simulink library "mympclib"  (R2020a)
settings: Solver=VariableStepAuto  StartTime=0.0  StopTime=10.0  RelTol=1e-3
undefined symbols (not defined in the file): params, sysm, Ts
(part 1 of 2)
settings Model: Creator=kohei  LastModifiedBy=kohei

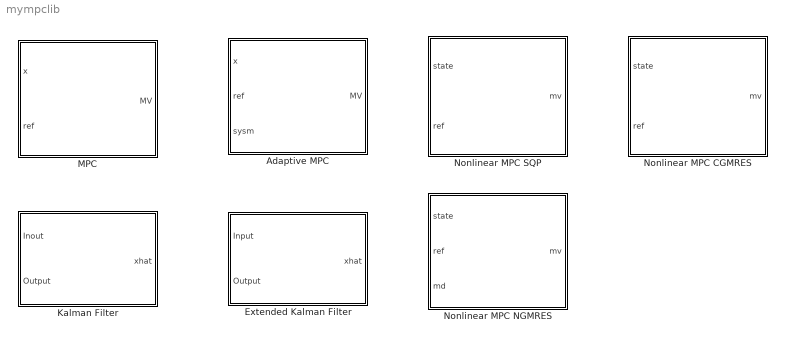
== system mympclib ==
  Adaptive MPC : Subsystem  TreatAsAtomicUnit=on  mask(Adaptive Model Predictive Control){params=params, numState=1, numRef=1, numMV=1, Ts=Ts, enableDist=off, numDist=1, enableSlack=off, enableStatus=off, enableMVseq=off}
      mask prompts: params "MPC Parameters"; numState "Dimension of State"; numRef "Dimension of Reference"; numMV "Dimension of Input"; Ts "Sampling time"; enableDist "Enable Disturbance Input"; numDist "Dimension of Disturbance"; enableSlack "Enable Slack Output"; enableStatus "Enable Status Output"; enableMVseq "Enable MVseq Output"
      mask help:
      | This is the Adaptive MPC (AMPC) Controller.
      | AMPC calculates the QP problem based on the linear plant model.
      | If you want to see the description, please push the help button.
      mask init:
      | numDist = initMaskPortMPC(numDist,enableDist,enableSlack,enableStatus,enableMVseq,'Adaptive MPC');
      | [params,~] = initMaskMPC(params,[],numState,numRef,numMV,numDist,'Adaptive MPC');
      | index = numState*params.PredictiveHorizon;
      | index2 = numMV*params.ControlHorizon;
      | index3 = numRef*params.PredictiveHorizon;
      | index4 = numMV*params.ControlHorizon+1;
      | index5 = 4*(numMV*params.ControlHorizon)+2*(numRef*params.PredictiveHorizon)+1;
      mask Help:
      | This block is the Adaptive MPC Controller.
      | AMPC calculates the QP problem based on the linear plant model.
      | 
      | >>Optimization formulation
      | -------------------------------------------------------------------------------------------------------------------------------------------------------------------
      | This MPC is formulated based on the next QP optimization.
      | 
      | J = 0.5 * ( (y - yref)'*Q*(y - yref) + du'*R*du + rho*slack^2 )
      | 
      | Subject to :
      | umin <= u <= umax
      | dumin <= du <= dumax
      | ymin - slack*vmin <= y <= ymax + slack*vmax
      | skack >= 0
      | 
      | One slack varable is introduced for relaxing the output constraint.
      | The vmin and vmax are the tunable parameter for relaxation which is able to specified by MPC parameter structure as "params.softConstRelaxation".
      | Please read the " Details of the parameter sturucture "params" and "sysm" ".
      | -------------------------------------------------------------------------------------------------------------------------------------------------------------------
      | 
      | >> Model Structure
      | -------------------------------------------------------------------------------------------------------------------------------------------------------------------
      | This block supports the discrete plant system as shown bellow:
      | Uppercase is indicated the Nominal value, Lowercase with 'd' suffix is indicated the perturbation.
      | 
      | State : x = X + dx
      | MV : u = U + du
      | Measurement Disturbance(MD) : md = MD + dmd
      | Output Value : y = Y +dy (dy = C*dx)
      | 
      | Model formulation :
      | dx(k+1) = A*dx(k)+ B*du(k) + Bd*dmd(k) + f0
      | y(K) = C*dx(K) + Y
      | 
      | Note : The direct feedthrough term "D" is not considered in this system.
      |           "f0" is the nominal value of the system at the operation point.
      | 
      | The plant model is streamed from the Input port "sysm" which is the Bus signal.
      | You need to define the Bus object named "sysBus" which includes A, B, Bd, C, f0 vector/matrix and the operation point of state, input, disturbance and output.
      | -------------------------------------------------------------------------------------------------------------------------------------------------------------------
      | 
      | >>Parameter
      | -------------------------------------------------------------------------------------------------------------------------------------------------------------------
      | The MPC parameter must be defined as structure variable.
      | And you must need to clarify the each dimension of "state", "ref", and "Input" and the Sampling time through mask dialog.
      | 
      | This block has four input ports "state", "ref", "md" and "sysm".
      | Where "n" is the order of state, "l" is the order of output value (OV), "m" is the order of manipulated variable (MV) and "nd" is the order of measurement disturbance (MD).
      | "state" : State variable of plant model (n×1)
      | "ref" : Reference for OV  (l×1)
      | "md" : Measurement Disturbance (nd×1)
      | "sysm" : Bus signal which includes the predictive model. The structuer of the Bus object is shown bellow :
      | 
      | sysm.A : A matrix
      | sysm.B : B matrix for MV
      | sysm.Bd : B matrix for MD
      | sysm.C : C matrix
      | sysm.U : Operation point of MV, Defalt : zeros(m,1)
      | sysm.MD : Operation point of MD, Default : zeros(nd,1)
      | sysm.Y : Operation point of OV, Default : zeros(l,1)
      | sysm.X : Operation point of state, Default : zeros(n,1)
      | sysm.f0: Operation point of system, Default : zeros(n,1)
      | 
      | You can create a Bus object automatically by uisng the API "createSysBusObject".
      | The API has four arguments 'n, m, nd, l'.
      | Example :
      | >sysBus = createSysBusObject(n,m,nd,l)
      | 
      | The output is four "mv" , "slack", "status" and "mvseq".
      | "mv" : Manipulated Variable which is optimized by MPC. (m×1)
      | "slack" : Slack variable for softening OV constrain. This value must be grater than 0 (>= 0).
      |              If the value is grater than 0, the OV constraint is softed to avoid infeasibe.
      | "status" : Status is for seeing whether or not feasible . If the value is "1", it means feasible, on the other hand the value is 0, it means infeasible.
      |                When the status is "0", the MPC applies a last MV for current step.
      | "mvseq": Sequence value of MV for futuer
      | -------------------------------------------------------------------------------------------------------------------------------------------------------------------
      | 
      | >>Solver
      | -------------------------------------------------------------------------------------------------------------------------------------------------------------------
      | You can choose two types solver for solving the QP.
      | First is the "Active set".
      | Second is the "Interior Point Method".
      | 
      | The Active set is appropriate to optimization class for small or middle size.
      | The Interior Point Method is appropriate to optimization class for large size.
      | 
      | Both default max iteration number is 50.
      | -------------------------------------------------------------------------------------------------------------------------------------------------------------------
      | 
      | >>Details of the parameter sturucture "params" and "sysm"
      | -------------------------------------------------------------------------------------------------------------------------------------------------------------------
      | The MPC parameter sturucture "params" must be configured as shown bellow :
      | Where "n" is the order of state, "l" is the order of OV, "m" is the order of MV and the "nd" is the order of MD.
      | 
      | params.Q : Weight of OV (l×l) , Default : Unit matrix
      | params.R : Weight of MV (m×m), Default : Unit matrix
      | params.PredictiveHorizon : Predictive horizon (Scalar), Default : 10
      | params.Controlhorizon : Control Horizon (Scalar), Default : 5
      | params.MV_max : MV max (m×1), Default : 999
      | params.MV_min : MV min (m×1), Default :  -999
      | params.dMV_max : Rate of MV max (m×1), Default : 999
      | params.dMV_min : Rate of MV min(m×1), Default : -999
      | params.OV_max : Rate of OV max (l×1), Default : 999
      | params.OV_min : Rate of OV min (l×1), Default : -999
      | params.rho : Weight of slack variable (Scalar), Default : 10^4
      | params.softConstRelaxation : Constant for OV relaxation by slack variable (l×1), Default : ones(l,1)
      | params.MV_scalefactor : Scale gain for MV (m×1), Default : ones(m,1)
      | params.OV_scalefactor : Scale gain for OV (l×1), Default : ones(m,1)
      | params.MD_scalefactor : Scale gain for MD (nd×1), Default : ones(m,1)
      | params.initialconditionMV : Initial value for MV (m×1), Default : ones(m,1)
      | params.SolverType :Scalar 1:= Active Set, 2:= Interior Point Method, Default : 1 (Active set)
      | params.IterationMax : Max iteration number of the QP solver, Default : 50
      | -------------------------------------------------------------------------------------------------------------------------------------------------------------------
      | 
      | >>Code generation
      | -------------------------------------------------------------------------------------------------------------------------------------------------------------------
      | Yes, support. If you have Simulink Coder and Embedded Coder, the implementation code can be generated from this block.
      | -------------------------------------------------------------------------------------------------------------------------------------------------------------------
      mask Callback enableDist:
      | enab = get_param(gcb,'enableDist');
      | 
      | % Set the 'MaskVisibilities' property for each parameters
      | if strcmp(enab,'on')
      |     set_param(gcb,'MaskVisibilities',{'on','on','on','on','on','on','on','on','on','on'});
      | else
      |     set_param(gcb,'MaskVisibilities',{'on','on','on','on','on','on','off','on','on','on'});
      | end
      mask Display:
      | fprintf('Adaptive MPC')
      | port_label('Output', 1, 'mv')
      | port_label('Input', 1, 'state')
      | port_label('Input', 2, 'ref')
      | port_label('Input', 3, 'sysm')
  Extended Kalman Filter : Subsystem  TreatAsAtomicUnit=on  mask(Extended Kalman filter){stateFunction=0, jacobianStateFunction=0, measurementFunction=0, jacobianMeasurmentFunction=0, Bv=0, Q=0, R=0, xhat0=0, P0=0, Ts=0, numState=0, numOutput=0, enableP=off, enableG=off}
      mask prompts: stateFunction "State Function"; jacobianStateFunction "Jacobian for the State Function"; measurementFunction "Measurment Function"; jacobianMeasurmentFunction "Jacobian for the Measurement Function"; Bv "Matrix for System noise v"; Q "Covariance matrix Q for system noise v"; R "Covariance matrix R for measurement noise w"; xhat0 "Initial value for xhat which is column vector"; P0 "Initial value for covariance matrix P"; Ts "Sampling time Ts"; numState "Order of state"; numOutput "Order of output"; enableP "Enable Covariance Marix output"; enableG "Enable Kalman Gain Matrix"
      mask help: This is the Extended Kalman filter(EKF) block.
      mask init:
      | p = initMaskEKF(stateFunction,measurementFunction,jacobianStateFunction,jacobianMeasurmentFunction);
      | initMaskPortKF(enableP,enableG,'EKF')
      mask Help:
      | This is the Extended Kalman filter(EKF) block.
      | Some parametrs are set through the mask diagram.
      | This block has two inputs named "Input" and "Output".
      | And it has three outputs named "xhat (Estimated state)", "P (Covariance matrix )" and "G (Kalman gain matrix )".
      | 
      | Support Formulation of EKF :
      | x(k+1) = f(x(k),u(k)) + Bv*v(k)
      | y(k) = h(x(k),u(k)) + w(k)
      | 
      | n : Order of state
      | m : Order of input
      | l : Order of output
      | 
      | f : Nonlinear dynamics function (n,1)
      | h : Nonlinear measurement function (l,1)
      | Bv : Gain matrix Bv for system noise v (n,n)
      | x : State (n,1)
      | u : Input (m,1)
      | v: System noise (n,1)
      | y : Output (l,1)
      | w : Measurement noise (l,1)
      | 
      | You need to prepare four MATLAB function and put them on the current folder or the MATLAB path.
      | Kind of the MATLAB function :
      | 
      | >Nonlinear discrete state function
      | 
      | >Jacobian of the Nonlinear state function about the state x with operate conditions x0 and u0.
      | 
      | >Nonlinear measurement function
      | 
      | >Jacobian of the Nonlinear measurement function about the state x with operate conditions x0 and u0.
      | 
      | Where, the above functions must be accepted three arguments x(state), u(input) and Ts(sampling time), and one output.
      | The order of three arguments has to be put as state, input and sampling time such like a below:
      | 
      | function out = fcn(x, u, Ts)
      | 
      | You have to set these function names through this mask dialog as the character array  by using sigle quotation.
      mask Display:
      | fprintf('Extended\n Kalman Filter')
      | port_label('Output', 1, 'xhat')
      | port_label('Input', 1, 'Input')
      | port_label('Input', 2, 'Output')
  Kalman Filter : Subsystem  TreatAsAtomicUnit=on  mask(Kalman filter){A=0, Bu=0, Bv=0, C=0, Q=0, R=0, xhat0=0, P0=0, Ts=0, enableP=off, enableG=off}
      mask prompts: A "System matrix A"; Bu "Input matrix Bu"; Bv "System noise matrix Bv"; C "Measurement matrix C"; Q "Covariance matrix for System noise v"; R "Covariance matrix for Measurement noise w"; xhat0 "Initial value for xhat which is column vector"; P0 "Initial value for covariance matrix P"; Ts "Sampling time Ts"; enableP "Enable Covariance Marix output"; enableG "Enable Kalman Gain Matrix"
      mask help: This is the LTI Kalman filter block.
      mask init:
      | initMaskPortKF(enableP,enableG,'KF')
      mask Help:
      | This is the LTI Kalman filter block.
      | All parametrs are set through the mask diagram.
      | This block has two inputs named "Input" and "Output".
      | And it has three outputs named "xhat (Estimated state)", "P (Covariance matrix )" and "G (Kalman gain matrix )".
      | 
      | Support Formulation of Kalman filter :
      | x(k+1) = A*x(k) + Bu*u(k) + Bv*v(k)
      | y(k) = C*x(k) + w(k)
      | 
      | A : System matrix A for state
      | Bu : System matrix Bu for input u
      | Bv : Gain matrix Bv for system noise v
      | C : System matrix C for output
      | x : State
      | u : Input
      | v : System noise
      | y : Output
      | w : Measurement noise
      mask Display:
      | fprintf('Kamlman Filter')
      | port_label('Output', 1, 'xhat')
      | port_label('Input', 1, 'Input')
      | port_label('Input', 2, 'Output')
  MPC : Subsystem  TreatAsAtomicUnit=on  mask(Model Predictive control){params=params, sysm=sysm, numState=1, numRef=1, numMV=1, Ts=Ts, enableDist=off, numDist=1, enableSlack=off, enableStatus=off, enableMVseq=off}
      mask prompts: params "MPC Parameters"; sysm "Control system"; numState "Dimension of State"; numRef "Dimension of Reference"; numMV "Dimension of MV"; Ts "Sampling time"; enableDist "Enable Disturbance Input"; numDist "Dimension of Disturbance"; enableSlack "Enable Slack Output"; enableStatus "Enable Status Output"; enableMVseq "Enable MVseq Output"
      mask help:
      | This is the MPC Controller.
      | MPC calculates the QP problem based on the linear plant model.
      | If you want to see the description, please push the help button.
      mask init:
      | numDist = initMaskPortMPC(numDist,enableDist,enableSlack,enableStatus,enableMVseq,'MPC');
      | [params,sysm] = initMaskMPC(params,sysm,numState,numRef,numMV,numDist,'MPC');
      | index = numState*params.PredictiveHorizon;
      | index2 = numMV*params.ControlHorizon;
      | index3 = numRef*params.PredictiveHorizon;
      | index4 = numMV*params.ControlHorizon+1;
      | index5 = 4*(numMV*params.ControlHorizon)+2*(numRef*params.PredictiveHorizon)+1;
      mask Help:
      | This block is the MPC Controller.
      | MPC calculates the QP problem based on the linear plant model.
      | 
      | >>Optimization formulation
      | -------------------------------------------------------------------------------------------------------------------------------------------------------------------
      | This MPC is formulated based on the next QP optimization.
      | 
      | J = 0.5 * ( (y - yref)'*Q*(y - yref) + du'*R*du + rho*slack^2 )
      | 
      | Subject to :
      | umin <= u <= umax
      | dumin <= du <= dumax
      | ymin - slack*vmin <= y <= ymax + slack*vmax
      | skack >= 0
      | 
      | One slack varable is introduced for releaxing the output constraint.
      | The vmin and vmax are tunable parameters for relaxation which are specified by the MPC parameter structure as "params.softConstRelaxation".
      | Please read the " Details of the parameter sturucture "params" and "sysm" ".
      | -------------------------------------------------------------------------------------------------------------------------------------------------------------------
      | 
      | 
      | >> Model Structure
      | -------------------------------------------------------------------------------------------------------------------------------------------------------------------
      | This block supports the discrete plant system as shown bellow:
      | Uppercase is indicated the Nominal value, Lowercase with 'd' suffix is indicated the perturbation.
      | 
      | State : x = X + dx
      | MV : u = U + du
      | Measurement Disturbance(MD) : md = MD + dmd
      | Output Value : y = Y +dy (dy = C*dx)
      | 
      | Model formulation :
      | dx(k+1) = A*dx(k)+ B*du(k) + Bd*dmd(k) + f0
      | y(K) = C*dx(K) + Y
      | 
      | Note : The direct feedthrough term "D" is not considered in this system.
      |           "f0" is the nominal value of the system at the operation point.
      | -------------------------------------------------------------------------------------------------------------------------------------------------------------------
      | 
      | 
      | >>Parameter
      | -------------------------------------------------------------------------------------------------------------------------------------------------------------------
      | The MPC parameter and the Control system must be defined as a structure variable.
      | The Sampling time must be set through mask dialog.
      | 
      | This block has three input ports "state", "ref" and "md".
      | Where, "n" is the order of state, "l" is the order of Output value (OV),  "m" is the order of Manipulated variable (MV) and "nd" is the order of measurment disturbance (MD).
      | "state" : State variable of plant model (n×1)
      | "ref" : Reference for OV  (l×1)
      | "md" : Measurement Disturbance (nd×1)
      | 
      | The output is three "mv" , "slack" and "status".
      | "MV" : Manipulated Variable which is optimized by MPC. (m×1)
      | "slack" : Slack variable for softening OV constrain. This value must be grater than 0 (>= 0).
      |              If the value is grater than 0, the OV constraint is softed to avoid infeasibe.
      | "status" : Status is for seeing whether or not feasible. If the value is "1", it means feasible, on the other hand the value is "0", it means infeasible.
      |                When the status is "0", the MPC applies a last MV for current step.
      | "mvseq": Sequence value of MV for futuer
      | -------------------------------------------------------------------------------------------------------------------------------------------------------------------
      | 
      | >>Solver
      | -------------------------------------------------------------------------------------------------------------------------------------------------------------------
      | You can choose two types solver for solving the QP.
      | First is the "Active set".
      | Second is the "Interior Point Method".
      | 
      | The Active set is appropriate to optimization class for small or middle size.
      | The Interior Point Method is appropriate to optimization class for large size.
      | 
      | Both default max iteration number is 50.
      | -------------------------------------------------------------------------------------------------------------------------------------------------------------------
      | 
      | >>Details of the parameter sturucture "params" and "sysm"
      | -------------------------------------------------------------------------------------------------------------------------------------------------------------------
      | The MPC parameter sturucture "params" must be configured as shown bellow :
      | Where the "n" is the order of state, "l" is the order of OV, "m" is the order of MV and the "nd" is the order of MD.
      | 
      | params.Q : Weight of OV (l×l) , Default : Unit matrix
      | params.R : Weight of MV (m×m), Default : Unit matrix
      | params.PredictiveHorizon : Predictive horizon (Scalar), Default : 10
      | params.Controlhorizon : Control Horizon (Scalar), Default : 5
      | params.MV_max : MV max (m×1), Default : 999
      | params.MV_min : MV min (m×1), Default :  -999
      | params.dMV_max : Rate of MV max (m×1), Default : 999
      | params.dMV_min : Rate of MV min(m×1), Default : -999
      | params.OV_max : Rate of OV max (l×1), Default : 999
      | params.OV_min : Rate of OV min (l×1), Default : -999
      | params.rho : Weight of slack variable (Scalar), Default : 10^4
      | params.softConstRelaxation : Constant for OV relaxation by slack variable (l×1), Default : ones(l,1)
      | params.MV_scalefactor : Scale gain for MV (m×1), Default : ones(m,1)
      | params.OV_scalefactor : Scale gain for OV (l×1), Default : ones(m,1)
      | params.MD_scalefactor : Scale gain for MD (nd×1), Default : ones(m,1)
      | params.initialconditionMV : Initial value for MV (m×1), Default : ones(m,1)
      | params.SolverType :Scalar, 1:= Active Set, 2:= Interior Point Method, Default : 1 (Active set)
      | params.IterationMax : Max iteration number of the QP solver, Default : 50
      | 
      | The Control system sturucture "syms" must be includes bellow items :
      | sysm.A : A matrix
      | sysm.B : B matrix for MV
      | sysm.Bd : B matrix for MD
      | sysm.C : C matrix
      | sysm.U : Operation point of MV, Defalt : zeros(m,1)
      | sysm.MD : Operation point of MD, Default : zeros(nd,1)
      | sysm.Y : Operation point of OV, Default : zeros(l,1)
      | sysm.X : Operation point of state, Default : zeros(n,1)
      | sysm.f0: Operation point of system, Default : zeros(n,1)
      | -------------------------------------------------------------------------------------------------------------------------------------------------------------------
      | 
      | >>Code generation
      | -------------------------------------------------------------------------------------------------------------------------------------------------------------------
      | Yes, support. If you have Simulink Coder and Embedded Coder, the implementation code can be generated from this block.
      | -------------------------------------------------------------------------------------------------------------------------------------------------------------------
      mask Callback enableDist:
      | enab = get_param(gcb,'enableDist');
      | 
      | % Set the 'MaskVisibilities' property for each parameters
      | if strcmp(enab,'on')
      |     set_param(gcb,'MaskVisibilities',{'on','on','on','on','on','on','on','on','on','on','on'});
      | else
      |     set_param(gcb,'MaskVisibilities',{'on','on','on','on','on','on','on','off','on','on','on'});
      | end
      mask Display:
      | fprintf('MPC')
      | port_label('Output', 1, 'mv')
      | port_label('Input', 1, 'state')
      | port_label('Input', 2, 'ref')
  Nonlinear MPC CGMRES : Subsystem  TreatAsAtomicUnit=on  mask(Nonlinear Model Predictive Control){params=params, nx=1, nmv=1, ns=1, nL=1, Ts=Ts, enableDist=off, nd=0, enableStatus=off, enableYseq=off, enableFnorm=off}
      mask prompts: params "MPC Parameters"; nx "Number of state"; nmv "Number of mv"; ns "Number of Slack"; nL "Number of Lagrange variable for constraint"; Ts "Sampling time"; enableDist "Enable Disturbance Input"; nd "Dimension of Disturbance"; enableStatus "Enable Status Output"; enableYseq "Enable Sequence Output"; enableFnorm "Enable F norm Output"
      mask help:
      | This is the NMPC Controller.
      | Calculate the Optimal Control Problem by using C/GMRES.
      | If you want to see the description, please push the help button.
      mask init:
      | nd = initMaskPortNMPC(nd,enableDist,[],enableStatus,enableYseq,enableFnorm,'CGMRES');
      | nyseq = [nx,params.divideNumber];
      | params = initMaskNMPC(params,nx,[],nmv,ns,nL,Ts,'CGMRES');
      mask Help:
      | This block is the Nonlinear MPC Controller.
      | Calculate the Optimal Control Problem by using C/GMRES.
      | 
      | >>Optimization formulation
      | -------------------------------------------------------------------------------------------------------------------------------------------------------------------
      | This MPC is formulated based on the next formulation.
      | 
      | J = Phi(x(tf),tf) + sum(L(x(t),u(t),t))  t = t0 to tf
      | Terminate Function : Phi(x(tf),tf) = x(tf)' *Qf*x(tf) note : tf is the time at the edge of prediction time
      | Stage cost function : L(x(t),u(t),t) = x(t)'*Q*x(t) + u(t)'*R*u(t)
      | 
      | Subject to :
      | xdot = f(x(t),u(t),t)
      | x(0) = x0
      | Ceq(x(t),u(t),t) = 0
      | Cinq(x(t),u(t),t) < 0
      | 
      | In the C/GMRES, you can introduce equality/inequality constraints.
      | In paticluar, inequality constraint can be considered by introducing slack variable or barrier function.
      | -------------------------------------------------------------------------------------------------------------------------------------------------------------------
      | 
      | 
      | >> Model Structure
      | -------------------------------------------------------------------------------------------------------------------------------------------------------------------
      | This block supports the continuous nonlinear plant system as shown bellow:
      | 
      | Model formulation :
      | xdot(t) = f( x(t), u(t), d(k) )
      | 
      | The "f" is the state function which is defined by MATLAB Function.
      | -------------------------------------------------------------------------------------------------------------------------------------------------------------------
      | 
      | 
      | >>Parameter
      | -------------------------------------------------------------------------------------------------------------------------------------------------------------------
      | The MPC parameter must be defined as structure variable.
      | And you must need to clarify the each dimension of "State", "Manipulated variable (MV)",  Slack, Lagrange variable for constrant, and Sampling time through mask dialog.
      | 
      | This block has three input ports "state", "ref", and "md".
      | Where "n" is the order of state, "m" is the order of manipulated variable (MV) and "nd" is the order of measurement disturbance (MD).
      | "state" : State variable of plant model (n×1)
      | "ref" : Reference for OV  (n×1)
      | "md" : Measurement Disturbance (nd×1)
      | 
      | The output is two "mv" and "status".
      | "mv" : Manipulated Variable which is optimized by MPC. (m×1)
      | "status" : Status is for seeing whether or not feasible. If the value is "1", it means feasible, on the other hand the value is 0, it means infeasible.
      |                When the value equals "0", the MPC applies a last MV for current step.
      | "yseq" : yseq is the sequential output from plant model while predition horizon.
      | "F": L2 norm of the nonlinear algebraic vector.
      | -------------------------------------------------------------------------------------------------------------------------------------------------------------------
      | 
      | 
      | >>Solver
      | -------------------------------------------------------------------------------------------------------------------------------------------------------------------
      | NMPC (CGMRES) block is implemented by Continuous and GMRES method.
      | C/GMRES method is developed by Prof. Otsuka from Kyoto univ.
      | In this method, nonliner OCP problem is solved by introducing GMRES instead of using Newton method.
      | The GMRES calculates the rate of the input and it is integrated in each sampling time Ts such like u = u + du*Ts.
      | GMRES method is guarateed to converge under the order of Krylov Subspace which equals to the order of design variable.
      | Default max iteration number is same to the order of Krylov Subspace.
      | -------------------------------------------------------------------------------------------------------------------------------------------------------------------
      | 
      | 
      | >>Details of the parameter sturucture "params".
      | -------------------------------------------------------------------------------------------------------------------------------------------------------------------
      | The MPC parameter sturucture "params" must be configured as shown bellow :
      | Where "n" is the order of state, "m" is the order of MV, "ns" is the order of the slack variable and "nL" is the order of the Lagrange varibale for the constraint.
      | 
      | params.stateFunction : Function name for the state transition
      | params.jacobianTerminalFunction : Function name for the jacobian about terminate function
      | params.jacobianHamiltonianState : Function name for the jacobian of state about hamiltonian function
      | params.jacobianHamiltonianInput : Function name for the jacobian of input about hamiltonian function
      | params.Q : Weight of State (n×1) , Default : Unit vector
      | params.Qf : Weight of State at termination (n×1) , Default : Unit vector
      | params.R : Weight of MV (m×1), Default : Unit matrix
      | params.PredictiveTime : Predictive Time [s] (Scalar), Default : 1
      | params.divideNumber : Separation number for predictive time  (Scalar), Default : 10
      | params.raiseGain : Raise Gain for increasing the prediction time  (Scalar), Default : 1
      | params.MV_max : MV max (m×1), Default : 999
      | params.MV_min : MV min (m×1), Default :  -999
      | params.zeta : Decay parameter  (Scalar), Default : 1/Ts
      | params.h : Small constant value for calculate the difference equation (Scalar), Default : 1e-3
      | params.initialConditionInputs : Initial value for Input ((m+ns+nL)×1), Default : zeros((m+ns+nL),1)
      | params.IterationMax : Max iteration number of the solver (Scalar), Default : (m+ns+nL)*divideNumber
      | -------------------------------------------------------------------------------------------------------------------------------------------------------------------
      | 
      | 
      | >>Tips for using CGMRES
      | -------------------------------------------------------------------------------------------------------------------------------------------------------------------
      | CGMRES uses the function handle, state transition and each Jacobian function.
      | You must need to follow the formulation of each function.
      | 
      | "stateFunction" has 1 output and 3 inputs, State, Input and Measurement Disturbance (MD).
      | "jacobianTerminalFunction" has 1 output and 3 inputs State, Reference of state and MPC parameter structuer "params".
      | "jacobianHamiltonianState" has 1 output and 6 inputs State, Lagrange variable which is Co-state, Input, MD, Reference of state and MPC parameter structuer.
      | "jacobianHamiltonianInput" has 1 output and 6 inputs State, Lagrange variable which is Co-state, Input, MD, Reference of state and MPC parameter structuer.
      | 
      | In the CGMRES, you can use some parameters for tuning and stable to the optimization process.
      | Qf, Q, R are the weights for state at tf, state while t0 to tf, and input.
      | These parameters work to change the resposiveness of the closed loop system and stabilization.
      | 
      | The PredictiveTime and the divideNumber are also used to decide a entire performance of the MPC.
      | If you use a large predictive time, MPC looks ahead in distant future.
      | But the calculation cost may be imapct foy your application.
      | And the divideNumber is the paranter how many steps you insert while pretictive time.
      | For example, the predictive time is 1[s] and the divideNumber is 10, MPC calcaulate 10 steps while 1[s].
      | Thus, the divideNumber equals to the sampling time for the predictive process.
      | Therefore, you can set another sampling time for predictive process against to the contol sampling time Ts.
      | 
      | The "raiseGain" is the parameter for characterize the speed of increasing the predictive time.
      | In CGMRES, to avoid a failure of the optimization process at first step, the predictive time increases slowly as the first order delay.
      | G = predictive time / ((raiseGain-1)*s + 1)
      | Thus, if you uses a large raiseGain, the output is soon matched to the predictive time.
      | 
      | "zeta" is the key parameter for CGMRES.
      | In CGMRES, it solves the derivatial eqations dF = -zeta * F.
      | Where F is the nonliear algebraic equation and CGMRES keeps to F as zero.
      | If some disturbances or erros are involved into system, F deviates from zero.
      | Thus, zeta works to regurate to zero.
      | If you set a large value of zeta, you specify strictly decay rate to the process.
      | In reference, zeta is recommended to equal inverse of sampling time Ts.
      | -------------------------------------------------------------------------------------------------------------------------------------------------------------------
      | 
      | 
      | >>Code generation
      | -------------------------------------------------------------------------------------------------------------------------------------------------------------------
      | Yes, support. If you have Simulink Coder and Embedded Coder, the implementation code can be generated from this block.
      | -------------------------------------------------------------------------------------------------------------------------------------------------------------------
      mask Callback nd:
      | enab = get_param(gcb,'enableDist');
      | 
      | % Set the 'MaskVisibilities' property for each parameters
      | if strcmp(enab,'on')
      |     set_param(gcb,'MaskVisibilities',{'on','on','on','on','on','on','on','on','on','on','on'});
      | else
      |     set_param(gcb,'MaskVisibilities',{'on','on','on','on','on','on','on','off','on','on','on'});
      | end
      mask Display:
      | fprintf('Nonlinear MPC\nC/GMRES')
      | port_label('Output', 1, 'mv')
      | port_label('Input', 1, 'state')
      | port_label('Input', 2, 'ref')
  Nonlinear MPC NGMRES : Subsystem  TreatAsAtomicUnit=on  mask(Nonlinear Model Predictive Control){params=params, nx=1, nmv=1, ns=1, nL=1, Ts=1, enableDist=on, nd=1, enableYseq=off, enableFnorm=off}
      mask prompts: params "MPC Parameters"; nx "Number of state"; nmv "Number of mv"; ns "Number of Slack"; nL "Number of Lagrange variable"; Ts "Sampling time"; enableDist "Enable Disturbance Input"; nd "Dimension of Disturbance"; enableYseq "Enable  Sequence Output"; enableFnorm "Enable F norm Output"
      mask help:
      | This is the NMPC Controller.
      | Calculate the Optimal Control Problem by using Newton-GMRES(NGMRES) method.
      | If you want to see the description, please push the help button.
      mask init:
      | nd = initMaskPortNMPC(nd,enableDist,[],0,enableYseq,enableFnorm,'NGMRES');
      | nyseq = [nx,params.divideNumber];
      | params = initMaskNMPC(params,nx,[],nmv,ns,nL,Ts,'NGMRES');
      | u0 = repmat(params.initialConditionInputs,params.divideNumber,1);
      | du0 = zeros(length(params.initialConditionInputs)*params.divideNumber,1);
      mask Help:
      | This block is the Nonlinear MPC Controller.
      | Calculate the Optimal Control Problem by using Newton-GMRES method.
      | 
      | >>Optimization formulation
      | -------------------------------------------------------------------------------------------------------------------------------------------------------------------
      | This MPC is formulated based on the next formulation.
      | 
      | J = Phi(x(tf),tf) + sum(L(x(t),u(t),t))  t = t0 to tf
      | Terminate Function : Phi(x(tf),tf) = x(tf)' *Qf*x(tf) note : tf is the time at the edge of prediction time
      | Stage cost function : L(x(t),u(t),t) = x(t)'*Q*x(t) + u(t)'*R*u(t)
      | 
      | Subject to :
      | xdot = f(x(t),u(t),t)
      | x(0) = x0
      | Ceq(x(t),u(t),t) = 0
      | Cinq(x(t),u(t),t) < 0
      | 
      | In the Newton-GMRES, you can introduce equality/inequality constraints.
      | In paticluar, inequality constraint can be considered by introducing slack variable or barrier function.
      | -------------------------------------------------------------------------------------------------------------------------------------------------------------------
      | 
      | 
      | >> Model Structure
      | -------------------------------------------------------------------------------------------------------------------------------------------------------------------
      | This block supports the continuous nonlinear plant system as shown bellow:
      | 
      | Model formulation :
      | xdot(t) = f( x(t), u(t), d(k) )
      | 
      | The "f" is the state function which is defined by MATLAB Function.
      | -------------------------------------------------------------------------------------------------------------------------------------------------------------------
      | 
      | 
      | >>Parameter
      | -------------------------------------------------------------------------------------------------------------------------------------------------------------------
      | The MPC parameter must be defined as structure variable.
      | And you must need to clarify the each dimension of "State", "Manipulated variable (MV)",  Slack, Lagrange variable for constrant, and Sampling time through mask dialog.
      | 
      | This block has three input ports "state", "ref", and "md".
      | Where "n" is the order of state, "m" is the order of manipulated variable (MV) and "nd" is the order of measurement disturbance (MD).
      | "state" : State variable of plant model (n×1)
      | "ref" : Reference for OV  (n×1)
      | "md" : Measurement Disturbance (nd×1)
      | 
      | The output is two "mv" and "status".
      | "mv" : Manipulated Variable which is optimized by MPC. (m×1)
      | "yseq" : yseq is the sequential output from plant model while predition horizon.
      | "F": L2 norm of the nonlinear algebraic vector.
      | -------------------------------------------------------------------------------------------------------------------------------------------------------------------
      | 
      | 
      | >>Solver
      | -------------------------------------------------------------------------------------------------------------------------------------------------------------------
      | NMPC (NGMRES) block is implemented by Newton-GMRES method.
      | Newton-GMRES method is iteration solver based on the newton step.
      | In each interval, this tries to calculate a solution by GMRES innner loop and Newton step outer loop.
      | Thus, in some cases, you need to expence more time for solving a problem than CGMRES.
      | In this solver, default max iteration number of the outer loop is set as 5 and that of innerloop is same as Krylov subspace.
      | -------------------------------------------------------------------------------------------------------------------------------------------------------------------
      | 
      | 
      | >>Details of the parameter sturucture "params".
      | -------------------------------------------------------------------------------------------------------------------------------------------------------------------
      | The MPC parameter sturucture "params" must be configured as shown bellow :
      | Where "n" is the order of state, "m" is the order of MV, "ns" is the order of the slack variable and "nL" is the order of the Lagrange varibale for the constraint.
      | 
      | params.stateFunction : Function name for the state transition
      | params.jacobianTerminalFunction : Function name for the jacobian about terminate function
      | params.jacobianHamiltonianState : Function name for the jacobian of state about hamiltonian function
      | params.jacobianHamiltonianInput : Function name for the jacobian of input about hamiltonian function
      | params.Q : Weight of State (n×1) , Default : Unit vector
      | params.Qf : Weight of State at termination (n×1) , Default : Unit vector
      | params.R : Weight of MV (m×1), Default : Unit matrix
      | params.PredictiveTime : Predictive Time [s] (Scalar), Default : 1
      | params.divideNumber : Separation number for predictive time  (Scalar), Default : 10
      | params.raiseGain : Raise Gain for increasing the prediction time  (Scalar), Default : 1
      | params.MV_max : MV max (m×1), Default : 999
      | params.MV_min : MV min (m×1), Default :  -999
      | params.h : Small constant value for calculate the difference equation (Scalar), Default : 1e-3
      | params.initialConditionInputs : Initial value for Input ((m+ns+nL)×1), Default : zeros((m+ns+nL),1)
      | params.InnrerIterationMax : Max iteration number of the inner loop (GMRES) (Scalar), Default : Default : (m+ns+nL)*divideNumber
      | params.OuterIterationMax : Max iteration number of the inner loop (Newton-step) (Scalar), Default : 5
      | -------------------------------------------------------------------------------------------------------------------------------------------------------------------
      | 
      | 
      | >>Tips for using NGMRES
      | -------------------------------------------------------------------------------------------------------------------------------------------------------------------
      | NGMRES uses the function handle, state transition and each Jacobian function.
      | You must need to follow the formulation of each function.
      | 
      | "stateFunction" has 1 output and 3 inputs, State, Input and Measurement Disturbance (MD).
      | "jacobianTerminalFunction" has 1 output and 3 inputs State, Reference of state and MPC parameter structuer "params".
      | "jacobianHamiltonianState" has 1 output and 6 inputs State, Lagrange variable which is Co-state, Input, MD, Reference of state and MPC parameter structuer.
      | "jacobianHamiltonianInput" has 1 output and 6 inputs State, Lagrange variable which is Co-state, Input, MD, Reference of state and MPC parameter structuer.
      | 
      | In the NGMRES, you can use some parameters for tuning and stable to the optimization process.
      | Qf, Q, R are the weights for state at tf, state while t0 to tf, and input.
      | These parameters work to change the resposiveness of the closed loop system and stabilization.
      | 
      | The PredictiveTime and the divideNumber are also used to decide a entire performance of the MPC.
      | If you use a large predictive time, MPC looks ahead in distant future.
      | But the calculation cost may be imapct foy your application.
      | And the divideNumber is the paranter how many steps you insert while pretictive time.
      | For example, the predictive time is 1[s] and the divideNumber is 10, MPC calculate 10 steps while 1[s].
      | Thus, the divideNumber equals to the sampling time for the predictive process.
      | Therefore, you can set another sampling time for predictive process against to the contol sampling time Ts.
      | 
      | The "raiseGain" is the parameter for characterize the speed of increasing the predictive time.
      | In NGMRES, to avoid a failure of the optimization process at first step, the predictive time increases slowly as the first order delay.
      | G = predictive time / ((raiseGain-1)*s + 1)
      | Thus, if you uses a large raiseGain, the output is soon matched to the predictive time.
      | -------------------------------------------------------------------------------------------------------------------------------------------------------------------
      | 
      | 
      | >>Code generation
      | -------------------------------------------------------------------------------------------------------------------------------------------------------------------
      | Yes, support. If you have Simulink Coder and Embedded Coder, the implementation code can be generated from this block.
      | -------------------------------------------------------------------------------------------------------------------------------------------------------------------
      mask Callback nd:
      | enab = get_param(gcb,'enableDist');
      | 
      | % Set the 'MaskVisibilities' property for each parameters
      | if strcmp(enab,'on')
      |     set_param(gcb,'MaskVisibilities',{'on','on','on','on','on','on','on','on','on','on'});
      | else
      |     set_param(gcb,'MaskVisibilities',{'on','on','on','on','on','on','on','off','on','on'});
      | end
      mask Display:
      | fprintf('Nonlinear MPC\nN/GMRES')
      | port_label('Output', 1, 'mv')
      | port_label('Input', 1, 'state')
      | port_label('Input', 2, 'ref')
      | port_label('Input', 3, 'md')
  Nonlinear MPC SQP : Subsystem  TreatAsAtomicUnit=on  mask(Nonlinear Model Predictive Control){params=params, nx=[], ny=1, nu=1, Ts=Ts, enableDist=off, nd=0, enableSlack=off, enableStatus=off}
      mask prompts: params "MPC Parameters"; nx "Dimension of State"; ny "Dimension of Output"; nu "Dimension of Input"; Ts "Sampling time"; enableDist "Enable Disturbance Input"; nd "Dimension of Disturbance"; enableSlack "Enable Slack Output"; enableStatus "Enable Status Output"
      mask help:
      | This is the NMPC Controller.
      | Calculate the NP problem by using the fmincon solver with SQP.
      |
      | Note :
      | "fmincon" is a builtin command of the Optimization Toolbox.
      | You need to install this toolbox for run this block.
      |
      | If you want to see the description, please push the help button.
      mask init:
      | nd = initMaskPortNMPC(nd,enableDist,enableSlack,enableStatus,[],[],'SQP');
      | params = initMaskNMPC(params,nx,ny,nu,[],[],Ts,'SQP');
      | mv0 = params.initialconditionMV;
      | x0 = params.initialconditionState;
      | Hp = params.PredictiveHorizon;
      | Hc = params.ControlHorizon;
      | d0 = [kron(ones(Hc,1),mv0);0];
      mask Help:
      | This block is the Nonlinear MPC Controller.
      | Calculate the NP problem by using the fmincon solver with SQP.
      | Note : "fmincon" is a builtin command of the Optimization Toolbox. You need to install this toolbox for run this block.
      | 
      | >>Optimization formulation
      | -------------------------------------------------------------------------------------------------------------------------------------------------------------------
      | This MPC is formulated based on the next QP optimization.
      | 
      | J = 0.5 * ( (y - yref)'*Q*(y - yref) + u'*R*u + rho*slack^2 )
      | 
      | Subject to :
      | umin <= u <= umax
      | dumin <= du <= dumax
      | ymin - slack*vmin <= y <= ymax + slack*vmax
      | skack >= 0
      | 
      | One slack varable is introduced for relaxing the output constraint.
      | The vmin and vmax are the tunable parameter for relaxation which is able to specified by MPC parameter structure as "params.softConstRelaxation".
      | Please read the " Details of the parameter sturucture "params"' and "sysm" ".
      | -------------------------------------------------------------------------------------------------------------------------------------------------------------------
      | 
      | 
      | >> Model Structure
      | -------------------------------------------------------------------------------------------------------------------------------------------------------------------
      | This block supports the discrete nonlinear plant system as shown bellow:
      | 
      | Model formulation :
      | dx(k+1) = f( x(k), u(k) ,d(k) )
      | y(K) = h( x(k), u(k) )
      | 
      | The "f" is the state function and the "h" is the measurement function.
      | These are defined by MATLAB Function.
      | -------------------------------------------------------------------------------------------------------------------------------------------------------------------
      | 
      | >>Parameter
      | -------------------------------------------------------------------------------------------------------------------------------------------------------------------
      | The MPC parameter must be defined as structure variable.
      | And you must need to clarify the each dimension of "State", "Output", "Input" and Sampling time through mask dialog.
      | 
      | This block has three input ports "state", "ref", and "md".
      | Where "n" is the order of state, "l" is the order of output value (OV),  "m" is the order of manipulated variable (MV) and "nd" is the order of measurement disturbance (MD).
      | "state" : State variable of plant model (n×1)
      | "ref" : Reference for OV  (l×1)
      | "md" : Measurement Disturbance (nd×1)
      | 
      | The output is three "mv" , "slack", and "status".
      | "mv" : Manipulated Variable which is optimized by MPC. (m×1)
      | "slack" : Slack variable for softening OV constraint. This value must be grater than 0 (>= 0).
      |              If the value is grater than 0, the OV constraint is softed to avoid infeasibe solution.
      | "status" : Status is for seeing whether or not feasible. If the value is "1", it means feasible, on the other hand the value is 0, it means infeasible.
      |                When the value equals "0", the MPC applies a last MV for current step.
      | -------------------------------------------------------------------------------------------------------------------------------------------------------------------
      | 
      | >>Solver
      | -------------------------------------------------------------------------------------------------------------------------------------------------------------------
      | NMPC block is implemented by using the "fmincon".
      | And for solving NP problem, SQP algorithm is used.
      | The "fmincon" is builtin command of the Optimization Toolbox.
      | So, you need to install the toolbox in your machine.
      | Default max iteration number is 50 times.
      | -------------------------------------------------------------------------------------------------------------------------------------------------------------------
      | 
      | >>Details of the parameter sturucture "params".
      | -------------------------------------------------------------------------------------------------------------------------------------------------------------------
      | The MPC parameter sturucture "params" must be configured as shown bellow :
      | Where "n" is the order of state, "l" is the order of OV, "m" is the order of MV.
      | 
      | params.stateFunction : Function name for the state evolution
      | params.measurementFunction : Function name for the measurement
      | params.Q : Weight of OV (l×l) , Default : Unit matrix
      | params.R : Weight of MV (m×m), Default : Unit matrix
      | params.PredictiveHorizon : Predictive horizon (Scalar), Default : 10
      | params.Controlhorizon : Control Horizon (Scalar), Default : 5
      | params.MV_max : MV max (m×1), Default : 999
      | params.MV_min : MV min (m×1), Default :  -999
      | params.dMV_max : Rate of MV max (m×1), Default : 999
      | params.dMV_min : Rate of MV min(m×1), Default : -999
      | params.OV_max : Rate of OV max (l×1), Default : 999
      | params.OV_min : Rate of OV min (l×1), Default : -999
      | params.rho : Weight of slack variable (Scalar), Default : 10^4
      | params.softConstRelaxation : Constant for OV relaxation by slack variable (l×1), Default : ones(l,1)
      | params.MV_scalefactor : Scale gain for MV (m×1), Default : ones(m,1)
      | params.OV_scalefactor : Scale gain for OV (l×1), Default : ones(m,1)
      | params.initialconditionMV : Initial value for MV (m×1), Default : zeros(m,1)
      | params.initialconditionState : Initial value for State (n×1), Default : zeros(m,1)
      | params.IterationMax : Max iteration number of the solver, Default : 50
      | -------------------------------------------------------------------------------------------------------------------------------------------------------------------
      | 
      | >>Code generation
      | -------------------------------------------------------------------------------------------------------------------------------------------------------------------
      | Yes, support. If you have Simulink Coder and Embedded Coder, the implementation code can be generated from this block.
      | -------------------------------------------------------------------------------------------------------------------------------------------------------------------
      mask Callback enableDist:
      | enab = get_param(gcb,'enableDist');
      | 
      | % Set the 'MaskVisibilities' property for each parameters
      | if strcmp(enab,'on')
      |     set_param(gcb,'MaskVisibilities',{'on','on','on','on','on','on','on','on','on'});
      | else
      |     set_param(gcb,'MaskVisibilities',{'on','on','on','on','on','on','off','on','on'});
      | end
      mask Callback enableStatus:
      | enab = get_param(gcb,'enableDist');
      | 
      | % Set the 'MaskVisibilities' property for each parameters
      | if strcmp(enab,'on')
      |     set_param(gcb,'MaskVisibilities',{'on','on','on','on','on','on','on','on','on'});
      | else
      |     set_param(gcb,'MaskVisibilities',{'on','on','on','on','on','on','off','on','on'});
      | end
      mask Display:
      | fprintf('Nonlinear MPC\nSQP')
      | port_label('Output', 1, 'mv')
      | port_label('Input', 1, 'state')
      | port_label('Input', 2, 'ref')
